simulink model "Loadflow4"  (R2017a)
settings: Solver=ode1  StartTime=0.0  StopTime=2  FixedStep=Time_Step  MaxStep=50e-6  RelTol=1e-3
undefined symbols (not defined in the file): fb, L, R, R_grid1, R_grid2, Theta01, Theta02, Time_Step, Un, Vm_RMS1, Vm_RMS2, wb, X_grid1, X_grid2
libraries: powerlib x29, powerlib_meascontrol x2
settings Model: Creator=Frederic_Colas  LastModifiedBy=Frederic_Colas
settings DataIOCC: ReturnWorkspaceOutputs=on
settings DebuggingCC: UnconnectedInputMsg=none  UnconnectedOutputMsg=none  UnconnectedLineMsg=none
settings SFSimCC: SimUseLocalCustomCode=on
settings RTWCC: RTWUseLocalCustomCode=on

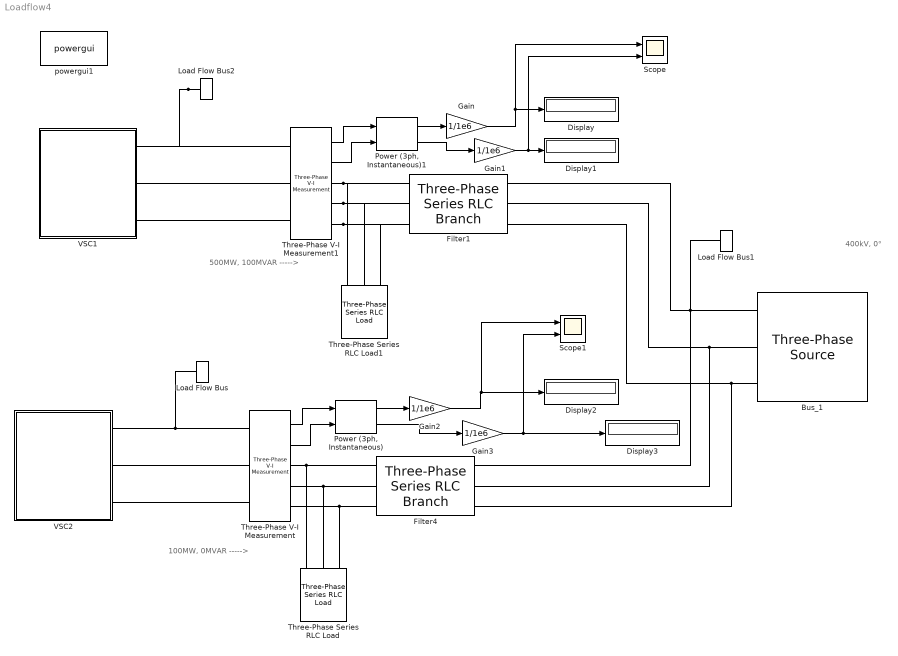
== system Loadflow4 ==
  note: 100MW, 0MVAR
      | ----->
  note: 400kV, 0°
  note: 500MW, 100MVAR
      | ----->
  Bus_1 : powerlib/Electrical Sources/Three-Phase Source  InternalConnection=Yg  VoltagePhases=off  Voltage=(400000)*1  PhaseAngle=0  Voltage_phases=[25e3 25e3 25e3]/sqrt(3)  PhaseAngles_phases=[0 -120 +120]  Frequency=fb  NonIdealSource=off  SpecifyImpedance=off  Resistance=0.8929  Inductance=16.58e-3  ShortCircuitLevel=100e6  BaseVoltage=25e3  XRratio=7  BusType=swing  Pref=10e3  Qref=0  Prefabc=[10e3, 10e3, 10e3]  Qrefabc=[0, 0, 0]  Qmin=-inf  Qmax=inf
  Display{,1..3} (4 alike) : Display
  Filter1 : powerlib/Elements/Three-Phase Series RLC Branch  LConnTagsString=A|B|C  RConnTagsString=A|B|C  BranchType=RL  Resistance=R_grid1  Inductance=X_grid1/wb  Capacitance=1e-6  Measurements=None
  Filter4 : powerlib/Elements/Three-Phase Series RLC Branch  LConnTagsString=A|B|C  RConnTagsString=A|B|C  BranchType=RL  Resistance=R_grid2  Inductance=X_grid2/wb  Capacitance=1e-6  Measurements=None
  Gain{,1..3} (4 alike) : Gain  Gain=1/1e6
  Load Flow Bus : powerlib/Measurements/Load Flow Bus  LConnTagsString=a  Phases=single  Connectors=on one side  ID=BUS_2  Vbase=Un  Vref=1  Vangle=0  VLF=0.9992  VLFb=1  VLFc=1  angleLF=-0.4572  angleLFb=0  angleLFc=0
  Load Flow Bus1 : powerlib/Measurements/Load Flow Bus  LConnTagsString=a  Phases=single  Connectors=on one side  ID=BUS_swing  Vbase=Un  Vref=1  Vangle=0  VLF=1  VLFb=1  VLFc=1  angleLF=0  angleLFb=0  angleLFc=0
  Load Flow Bus2 : powerlib/Measurements/Load Flow Bus  LConnTagsString=a  Phases=single  Connectors=on one side  ID=BUS_1  Vbase=Un  Vref=1  Vangle=0  VLF=1.005  VLFb=1  VLFc=1  angleLF=0.8865  angleLFb=0  angleLFc=0
  "Power (3ph, Instantaneous)" : powerlib_meascontrol/Measurements/Power (3ph, Instantaneous)
  "Power (3ph, Instantaneous)1" : powerlib_meascontrol/Measurements/Power (3ph, Instantaneous)
  Scope : Scope  NumInputPorts=2
  Scope1 : Scope  NumInputPorts=2
  Three-Phase Series RLC Load : powerlib/Elements/Three-Phase Series RLC Load  LConnTagsString=A|B|C  Configuration=Y (grounded)  NominalVoltage=400e3  Vabc=[1e3 1e3 1e3]  Vabcp=[1e3 1e3 1e3]  NominalFrequency=50  UnbalancedPower=off  ActivePower=200e6  InductivePower=0  CapacitivePower=0  Pabc=[10e3 9e3 11e3]  QLabc=[100 90 110]  QCabc=[100 90 110]  Pabcp=[10e3 9e3 11e3]  QLabcp=[100 90 110]  QCabcp=[100 90 110]  Measurements=None  LoadType=constant Z
  Three-Phase Series RLC Load1 : powerlib/Elements/Three-Phase Series RLC Load  LConnTagsString=A|B|C  Configuration=Y (grounded)  NominalVoltage=400e3  Vabc=[1e3 1e3 1e3]  Vabcp=[1e3 1e3 1e3]  NominalFrequency=50  UnbalancedPower=off  ActivePower=100e6  InductivePower=0  CapacitivePower=0  Pabc=[10e3 9e3 11e3]  QLabc=[100 90 110]  QCabc=[100 90 110]  Pabcp=[10e3 9e3 11e3]  QLabcp=[100 90 110]  QCabcp=[100 90 110]  Measurements=None  LoadType=constant Z
  Three-Phase V-I Measurement : powerlib/Measurements/Three-Phase V-I Measurement  VoltageMeasurement=phase-to-ground  SetLabelV=off  LabelV=Vabc  Vpu=off  VpuLL=off  CurrentMeasurement=yes  SetLabelI=off  LabelI=Iabc  Ipu=off  Pbase=100e6  Vbase=500e3  OutputType=Complex  PhasorSimulation=off  PSBequivalent=0
  Three-Phase V-I Measurement1 : powerlib/Measurements/Three-Phase V-I Measurement  VoltageMeasurement=phase-to-ground  SetLabelV=off  LabelV=Vabc  Vpu=off  VpuLL=off  CurrentMeasurement=yes  SetLabelI=off  LabelI=Iabc  Ipu=off  Pbase=100e6  Vbase=500e3  OutputType=Complex  PhasorSimulation=off  PSBequivalent=0
  VSC1 : Subsystem  mask{Un=Un, Vm_RMS=Vm_RMS1, Theta0=Theta01}
      mask prompts: Un "ph-ph Nominal voltage (V)"; Vm_RMS "Vm_RMS (V)"; Theta0 "angle  (deg)"
      mask init:
      | Theta0 = Theta0*pi/180;
  VSC2 : Subsystem  mask{Un=Un, Vm_RMS=Vm_RMS2, Theta0=Theta02}
      mask prompts: Un "ph-ph Nominal voltage (V)"; Vm_RMS "Vm_RMS (V)"; Theta0 "angle  (deg)"
      mask init:
      | Theta0 = Theta0*pi/180;
  powergui1 : powerlib/powergui  Priority=1  SimulationMode=Discrete  SampleTime=Time_Step  frequency=60  Iterations=50  frequencyindice=50  Pbase=1000000000  ErrMax=1e-06  UnitsV=kV  UnitsW=MW  buscounter=0  FunctionMessages=off  echomessages=off  EnableUseOfTLC=off  CurrentSourceSwitches=off  DisableSnubberDevices=off  DisableRonSwitches=off  DisableVfSwitches=off  DisplayEquations=off  AutomaticDiscreteSolvers=off  SolverType=Tustin/Backward Euler (TBE)  Interpol=off  ExternalGateDelay=off  methode=off  Ts=100  x0status=blocks  SPID=on  SwTol=0  HookPort=off  NonlinearTolerance=1e-4  nMaxIteration=100  ContinueOnMaxIteration=off  RestoreLinks=warning  ResistiveCurrentMeasurement=off  Frange=[0:2:500]  Ylog=off  Xlog=on  ShowGrid=off  save=off  variable=ZData  structure=0  ZoomFFT=off  StartTime=0.0  cycles=1  DisplayStyle=1  fundamental=60  FreqAxis=off  MaxFrequency=1000  frequencyindicesteady=1  RmsSteady=1  display=off
  wires:
  Three-Phase V-I Measurement/1 -> "Power (3ph, Instantaneous)"/1
  Three-Phase V-I Measurement/2 -> "Power (3ph, Instantaneous)"/2
  "Power (3ph, Instantaneous)"/1 -> Gain2/1
  "Power (3ph, Instantaneous)"/2 -> Gain3/1
  Three-Phase V-I Measurement1/2 -> "Power (3ph, Instantaneous)1"/2
  "Power (3ph, Instantaneous)1"/2 -> Gain1/1
  Three-Phase V-I Measurement1/1 -> "Power (3ph, Instantaneous)1"/1
  "Power (3ph, Instantaneous)1"/1 -> Gain/1
  Gain/1 -> Scope/1, Display/1
  Gain1/1 -> Scope/2, Display1/1
  Gain3/1 -> Scope1/2, Display3/1
  Gain2/1 -> Scope1/1, Display2/1
  connections:
  Three-Phase V-I Measurement/LConn1 -- VSC2/RConn1 -- Load Flow Bus/LConn1
  Three-Phase Series RLC Load/LConn1 -- Filter4/LConn1 -- Three-Phase V-I Measurement/RConn1
  Three-Phase Series RLC Load/LConn2 -- Filter4/LConn2 -- Three-Phase V-I Measurement/RConn2
  Three-Phase Series RLC Load/LConn3 -- Filter4/LConn3 -- Three-Phase V-I Measurement/RConn3
  Filter1/RConn2 -- Filter4/RConn2 -- Bus_1/RConn2
  Load Flow Bus1/LConn1 -- Filter4/RConn1 -- Filter1/RConn1 -- Bus_1/RConn1
  Filter1/RConn3 -- Filter4/RConn3 -- Bus_1/RConn3
  VSC2/RConn2 -- Three-Phase V-I Measurement/LConn2
  VSC2/RConn3 -- Three-Phase V-I Measurement/LConn3
  Three-Phase V-I Measurement1/RConn1 -- Filter1/LConn1 -- Three-Phase Series RLC Load1/LConn1
  Three-Phase V-I Measurement1/RConn3 -- Filter1/LConn3 -- Three-Phase Series RLC Load1/LConn3
  Load Flow Bus2/LConn1 -- VSC1/RConn1 -- Three-Phase V-I Measurement1/LConn1
  Three-Phase V-I Measurement1/RConn2 -- Filter1/LConn2 -- Three-Phase Series RLC Load1/LConn2
  VSC1/RConn2 -- Three-Phase V-I Measurement1/LConn2
  VSC1/RConn3 -- Three-Phase V-I Measurement1/LConn3

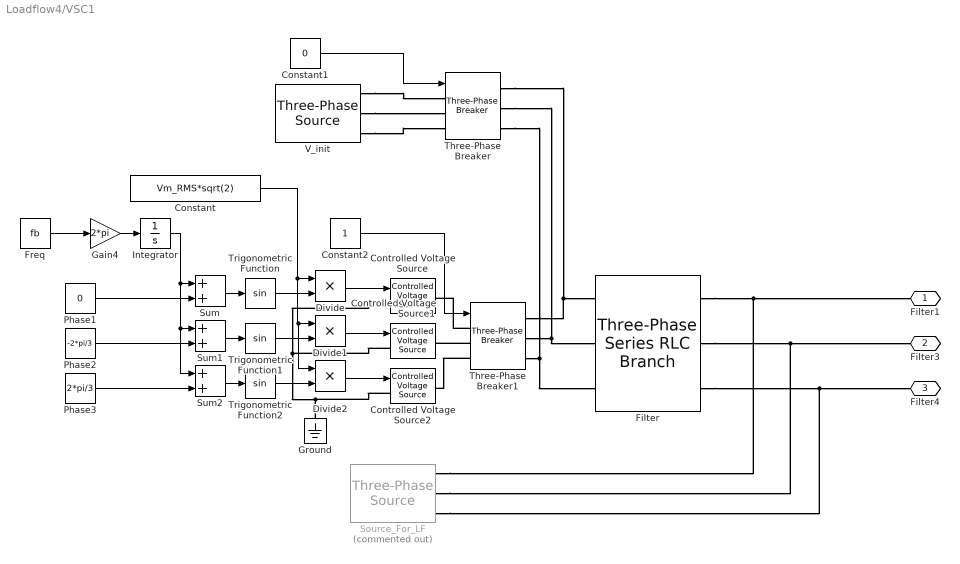
== system Loadflow4/VSC1 ==
  Constant : Constant  Value=Vm_RMS*sqrt(2)
  Constant1 : Constant  Value=0
  Constant2 : Constant
  Controlled Voltage Source : powerlib/Electrical Sources/Controlled Voltage Source  Initialize=off  Source_Type=AC  Amplitude=Vm_RMS*sqrt(2)  Phase=Theta0*180/pi  Frequency=fb  Measurements=None
  Controlled Voltage Source1 : powerlib/Electrical Sources/Controlled Voltage Source  Initialize=off  Source_Type=AC  Amplitude=Vm_RMS*sqrt(2)  Phase=Theta0*180/pi-2*pi/3  Frequency=fb  Measurements=None
  Controlled Voltage Source2 : powerlib/Electrical Sources/Controlled Voltage Source  Initialize=off  Source_Type=AC  Amplitude=Vm_RMS*sqrt(2)  Phase=Theta0*180/pi-4*pi/3  Frequency=fb  Measurements=None
  Divide : Product  Inputs=**
  Divide1 : Product  Inputs=**
  Divide2 : Product  Inputs=**
  Filter : powerlib/Elements/Three-Phase Series RLC Branch  LConnTagsString=A|B|C  RConnTagsString=A|B|C  BranchType=RL  Resistance=R  Inductance=L  Capacitance=1e-6  Measurements=None
  Freq : Constant  Value=fb
  Gain4 : Gain  Gain=2*pi
  Ground : powerlib/Elements/Ground  LConnTagsString=a
  Integrator : Integrator  InitialCondition=Theta0
  Phase1 : Constant  Value=0
  Phase2 : Constant  Value=-2*pi/3
  Phase3 : Constant  Value=2*pi/3
  Source_For_LF : powerlib/Electrical Sources/Three-Phase Source  Commented=on  InternalConnection=Yg  VoltagePhases=off  Voltage=(400000)*1.00545  PhaseAngle=0.88652  Voltage_phases=[25e3 25e3 25e3]/sqrt(3)  PhaseAngles_phases=[0 -120 +120]  Frequency=fb  NonIdealSource=off  SpecifyImpedance=off  Resistance=0.8929  Inductance=16.58e-3  ShortCircuitLevel=100e6  BaseVoltage=25e3  XRratio=7  BusType=PQ  Pref=500e6  Qref=100e6  Prefabc=[10e3, 10e3, 10e3]  Qrefabc=[0, 0, 0]  Qmin=-inf  Qmax=inf
  Sum : Sum
  Sum1 : Sum
  Sum2 : Sum
  Three-Phase Breaker : powerlib/Elements/Three-Phase Breaker  InitialState=closed  SwitchA=on  SwitchB=on  SwitchC=on  SwitchTimes="[1/60  5/60]"  External=on  BreakerResistance=0.0001  SnubberResistance=1e6  SnubberCapacitance=inf  Measurements=None
  Three-Phase Breaker1 : powerlib/Elements/Three-Phase Breaker  InitialState=open  SwitchA=on  SwitchB=on  SwitchC=on  SwitchTimes="[1/60  5/60]"  External=on  BreakerResistance=0.0001  SnubberResistance=1e6  SnubberCapacitance=inf  Measurements=None
  Trigonometric Function : Trigonometry
  Trigonometric Function1 : Trigonometry
  Trigonometric Function2 : Trigonometry
  V_init : powerlib/Electrical Sources/Three-Phase Source  InternalConnection=Yg  VoltagePhases=off  Voltage=Vm_RMS*sqrt(3)  PhaseAngle=Theta0*180/pi  Voltage_phases=[25e3 25e3 25e3]/sqrt(3)  PhaseAngles_phases=[0 -120 +120]  Frequency=fb  NonIdealSource=off  SpecifyImpedance=off  Resistance=0.8929  Inductance=16.58e-3  ShortCircuitLevel=100e6  BaseVoltage=25e3  XRratio=7  BusType=PQ  Pref=500e6  Qref=100e6  Prefabc=[10e3, 10e3, 10e3]  Qrefabc=[0, 0, 0]  Qmin=-inf  Qmax=inf
  Filter1 : PMIOPort  Side=Right
  Filter3 : PMIOPort  Port=2  Side=Right
  Filter4 : PMIOPort  Port=3  Side=Right
  wires:
  Constant/1 -> Divide2/1, Divide1/1, Divide/1
  Sum2/1 -> Trigonometric Function2/1
  Gain4/1 -> Integrator/1
  Freq/1 -> Gain4/1
  Divide1/1 -> Controlled Voltage Source1/1
  Divide2/1 -> Controlled Voltage Source2/1
  Phase1/1 -> Sum/2
  Trigonometric Function1/1 -> Divide1/2
  Sum1/1 -> Trigonometric Function1/1
  Integrator/1 -> Sum2/1, Sum1/1, Sum/1
  Phase2/1 -> Sum1/2
  Trigonometric Function2/1 -> Divide2/2
  Trigonometric Function/1 -> Divide/2
  Sum/1 -> Trigonometric Function/1
  Divide/1 -> Controlled Voltage Source/1
  Phase3/1 -> Sum2/2
  Constant1/1 -> Three-Phase Breaker/1
  Constant2/1 -> Three-Phase Breaker1/1
  connections:
  Filter/RConn1 -- Source_For_LF/RConn1 -- Filter1/RConn1
  Controlled Voltage Source1/LConn1 -- Controlled Voltage Source/LConn1 -- Controlled Voltage Source2/LConn1 -- Ground/LConn1
  Filter/RConn3 -- Source_For_LF/RConn3 -- Filter4/RConn1
  Filter/RConn2 -- Source_For_LF/RConn2 -- Filter3/RConn1
  Three-Phase Breaker/RConn1 -- Three-Phase Breaker1/RConn1 -- Filter/LConn1
  Three-Phase Breaker/RConn2 -- Filter/LConn2 -- Three-Phase Breaker1/RConn2
  Three-Phase Breaker/RConn3 -- Filter/LConn3 -- Three-Phase Breaker1/RConn3
  Three-Phase Breaker1/LConn2 -- Controlled Voltage Source1/RConn1
  Three-Phase Breaker1/LConn1 -- Controlled Voltage Source/RConn1
  Three-Phase Breaker1/LConn3 -- Controlled Voltage Source2/RConn1
  V_init/RConn2 -- Three-Phase Breaker/LConn2
  V_init/RConn1 -- Three-Phase Breaker/LConn1
  V_init/RConn3 -- Three-Phase Breaker/LConn3

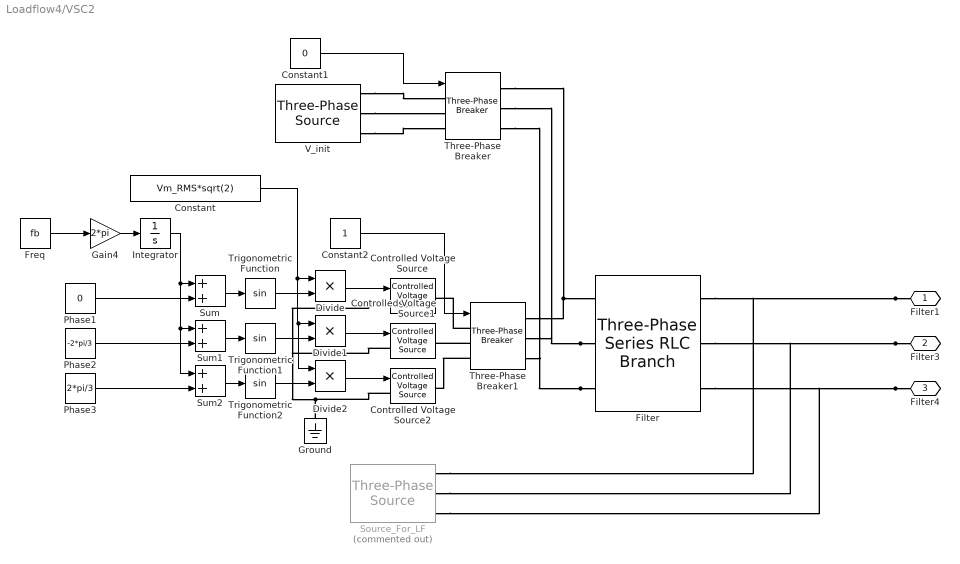
== system Loadflow4/VSC2 ==
  Constant : Constant  Value=Vm_RMS*sqrt(2)
  Constant1 : Constant  Value=0
  Constant2 : Constant
  Controlled Voltage Source : powerlib/Electrical Sources/Controlled Voltage Source  Initialize=off  Source_Type=AC  Amplitude=Vm_RMS*sqrt(2)  Phase=Theta0*180/pi  Frequency=fb  Measurements=None
  Controlled Voltage Source1 : powerlib/Electrical Sources/Controlled Voltage Source  Initialize=off  Source_Type=AC  Amplitude=Vm_RMS*sqrt(2)  Phase=Theta0*180/pi-2*pi/3  Frequency=fb  Measurements=None
  Controlled Voltage Source2 : powerlib/Electrical Sources/Controlled Voltage Source  Initialize=off  Source_Type=AC  Amplitude=Vm_RMS*sqrt(2)  Phase=Theta0*180/pi-4*pi/3  Frequency=fb  Measurements=None
  Divide : Product  Inputs=**
  Divide1 : Product  Inputs=**
  Divide2 : Product  Inputs=**
  Filter : powerlib/Elements/Three-Phase Series RLC Branch  LConnTagsString=A|B|C  RConnTagsString=A|B|C  BranchType=RL  Resistance=R  Inductance=L  Capacitance=1e-6  Measurements=None
  Freq : Constant  Value=fb
  Gain4 : Gain  Gain=2*pi
  Ground : powerlib/Elements/Ground  LConnTagsString=a
  Integrator : Integrator  InitialCondition=Theta0
  Phase1 : Constant  Value=0
  Phase2 : Constant  Value=-2*pi/3
  Phase3 : Constant  Value=2*pi/3
  Source_For_LF : powerlib/Electrical Sources/Three-Phase Source  Commented=on  InternalConnection=Yg  VoltagePhases=off  Voltage=(400000)*1.00545  PhaseAngle=0.88652  Voltage_phases=[25e3 25e3 25e3]/sqrt(3)  PhaseAngles_phases=[0 -120 +120]  Frequency=fb  NonIdealSource=off  SpecifyImpedance=off  Resistance=0.8929  Inductance=16.58e-3  ShortCircuitLevel=100e6  BaseVoltage=25e3  XRratio=7  BusType=PQ  Pref=500e6  Qref=100e6  Prefabc=[10e3, 10e3, 10e3]  Qrefabc=[0, 0, 0]  Qmin=-inf  Qmax=inf
  Sum : Sum
  Sum1 : Sum
  Sum2 : Sum
  Three-Phase Breaker : powerlib/Elements/Three-Phase Breaker  InitialState=closed  SwitchA=on  SwitchB=on  SwitchC=on  SwitchTimes="[1/60  5/60]"  External=on  BreakerResistance=0.0001  SnubberResistance=1e6  SnubberCapacitance=inf  Measurements=None
  Three-Phase Breaker1 : powerlib/Elements/Three-Phase Breaker  InitialState=open  SwitchA=on  SwitchB=on  SwitchC=on  SwitchTimes="[1/60  5/60]"  External=on  BreakerResistance=0.0001  SnubberResistance=1e6  SnubberCapacitance=inf  Measurements=None
  Trigonometric Function : Trigonometry
  Trigonometric Function1 : Trigonometry
  Trigonometric Function2 : Trigonometry
  V_init : powerlib/Electrical Sources/Three-Phase Source  InternalConnection=Yg  VoltagePhases=off  Voltage=Vm_RMS*sqrt(3)  PhaseAngle=Theta0*180/pi  Voltage_phases=[25e3 25e3 25e3]/sqrt(3)  PhaseAngles_phases=[0 -120 +120]  Frequency=fb  NonIdealSource=off  SpecifyImpedance=off  Resistance=0.8929  Inductance=16.58e-3  ShortCircuitLevel=100e6  BaseVoltage=25e3  XRratio=7  BusType=PQ  Pref=500e6  Qref=100e6  Prefabc=[10e3, 10e3, 10e3]  Qrefabc=[0, 0, 0]  Qmin=-inf  Qmax=inf
  Filter1 : PMIOPort  Side=Right
  Filter3 : PMIOPort  Port=2  Side=Right
  Filter4 : PMIOPort  Port=3  Side=Right
  wires:
  Constant2/1 -> Three-Phase Breaker1/1
  Constant1/1 -> Three-Phase Breaker/1
  Phase3/1 -> Sum2/2
  Divide/1 -> Controlled Voltage Source/1
  Sum/1 -> Trigonometric Function/1
  Trigonometric Function/1 -> Divide/2
  Trigonometric Function2/1 -> Divide2/2
  Phase2/1 -> Sum1/2
  Integrator/1 -> Sum/1, Sum1/1, Sum2/1
  Sum1/1 -> Trigonometric Function1/1
  Trigonometric Function1/1 -> Divide1/2
  Phase1/1 -> Sum/2
  Divide2/1 -> Controlled Voltage Source2/1
  Divide1/1 -> Controlled Voltage Source1/1
  Freq/1 -> Gain4/1
  Gain4/1 -> Integrator/1
  Sum2/1 -> Trigonometric Function2/1
  Constant/1 -> Divide/1, Divide1/1, Divide2/1
  connections:
  V_init/RConn3 -- Three-Phase Breaker/LConn3
  V_init/RConn1 -- Three-Phase Breaker/LConn1
  V_init/RConn2 -- Three-Phase Breaker/LConn2
  Three-Phase Breaker1/LConn3 -- Controlled Voltage Source2/RConn1
  Three-Phase Breaker1/LConn1 -- Controlled Voltage Source/RConn1
  Three-Phase Breaker1/LConn2 -- Controlled Voltage Source1/RConn1
  Filter/LConn3 -- Three-Phase Breaker/RConn3 -- Three-Phase Breaker1/RConn3
  Filter/LConn2 -- Three-Phase Breaker/RConn2 -- Three-Phase Breaker1/RConn2
  Three-Phase Breaker1/RConn1 -- Three-Phase Breaker/RConn1 -- Filter/LConn1
  Filter3/RConn1 -- Source_For_LF/RConn2 -- Filter/RConn2
  Filter4/RConn1 -- Source_For_LF/RConn3 -- Filter/RConn3
  Ground/LConn1 -- Controlled Voltage Source2/LConn1 -- Controlled Voltage Source/LConn1 -- Controlled Voltage Source1/LConn1
  Filter1/RConn1 -- Source_For_LF/RConn1 -- Filter/RConn1
